simulink model "simulink_sketch"  (R2025b)
settings: Solver=VariableStepAuto  StartTime=0.0  StopTime=5  FixedStep=1e-6  MaxStep=1e-5  RelTol=1e-4
values from neighbouring files (symbols this model uses):
  bb_Cb = 1e-4    (= 0.0001)    [Akobel.m]
  bb_L2 = 1e-3    (= 0.001)    [Akobel.m]
  bb_R2 = 0.1    [Akobel.m]
  bb_series_R = 0.01    [Akobel.m]
  boost_Cdc = 2200e-6    (= 0.0022)    [Akobel.m]
  boost_Fsw = 10000    [Akobel.m]
  boost_L1 = 200e-6    (= 0.0002)    [Akobel.m]
  boost_R1 = 0.5    [Akobel.m]
  cc_Ib_trim_max = 0.5    [Akobel.m]
  cc_Iff_max = 1    [Akobel.m]
  cc_Ki = 0.02    [Akobel.m]
  cc_Kp = 0.002    [Akobel.m]
  cc_Ts = 1e-3    (= 0.001)    [Akobel.m]
  cc_Vdc_ref = 150    [Akobel.m]
  grid_freq = 60    [Akobel.m]
  grid_Ls1 = 0.05    [Akobel.m]
  grid_Rs1 = 5    [Akobel.m]
  grid_Vrms_test = 30.3    [Akobel.m]
  mppt_dD = 0.001    [Akobel.m]
  mppt_Dold_init = 0.75    [Akobel.m]
  mppt_filter_alpha = 0.1    [Akobel.m]
  mppt_max_duty_step = 0.02    [Akobel.m]
  mppt_Ts = 0.1    [Akobel.m]
  mppt_Vdc_hyst = 15    [Akobel.m]
  mppt_Vdc_start_clamp = 220    [Akobel.m]
  mppt_Vdc_trip = 280    [Akobel.m]
  pv_Cpv = 1000e-6    (= 0.001)    [Akobel.m]
  pv_irradiance = 1000    [Akobel.m]
  pv_temperature = 25    [Akobel.m]
  pwm_dt_deadtime_frac = 0.02    [Akobel.m]
  Ts = 1e-6    (= 1e-06)    [Akobel.m]
  xfmr_L_pu = 0.08    [Akobel.m]
  xfmr_R_pu = 0.002    [Akobel.m]
  xfmr_Sn_test = 5000    [Akobel.m]
  xfmr_V_test = grid_Vrms_test    (= 30.3)    [Akobel.m]
undefined symbols (not defined in the file or in its folder): Ion, Lithium
libraries: spsSeriesRLCBranchLib x11, spsIGBTLib x3, spsVoltageMeasurementLib x3, spsThreePhaseTransformerTwoWindingsLib x2, spsThreePhaseVIMeasurementLib x2, spsabctodq0Lib x2, spsPVArrayLib x1, spsDiodeLib x1, spsPWMGeneratorDCDCLib x1, spsBatteryLib x1, spsCurrentMeasurementLib x1, slpidlib x1
settings Model: Creator=inspiredkhalid  LastModifiedBy=inspiredkhalid

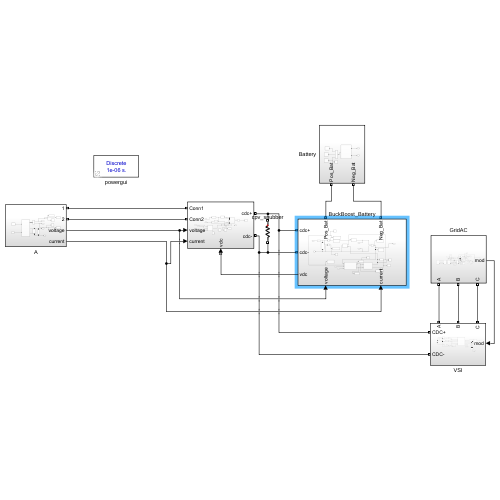
[thumbnail: Simulink's stored preview of the top-level diagram]
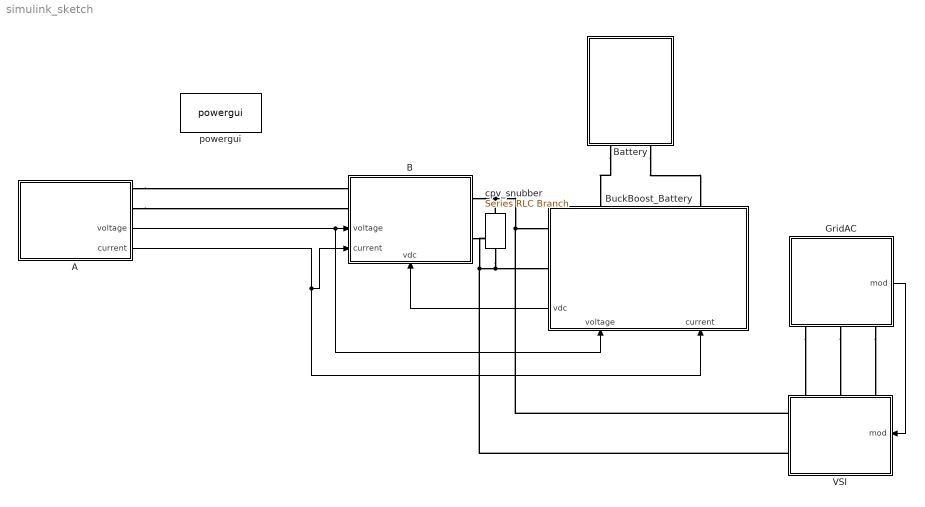
== system simulink_sketch ==
  A : Subsystem
      settings: PortSchema="{\"entries\":[{\"content\":{\"sides\":[{\"content\":{\"connectorIds\":[\"LConn1\",\"LConn2\",\"Out1\",\"Out2\"]},\"type\":\"ConnectorPlacement.EquallySpacedRectSide\",\"uuid\":\"f211f14f-7a8f-4763-b05c-a6f88137a125\"},{\"content\":{\"side\":\"RIGHT\"},\"type\":\"ConnectorPlacement.EquallySpacedRectSide\",\"uuid\":\"e9ab2bdb-56c2-498f-9900-91b8c83bb3bf\"},{\"content\":{\"side\":\"TOP\"},\"type\":\"ConnectorPlacement.EquallySpacedRectSide\",\"uuid\":\"9658df41-4415-4477-a305-d7a4a909d21d\"}]},\"type\":\"ConnectorPlacement.EquallySpacedConnector\",\"uuid\":\"93cd9b4f-abff-4e5b-becd-fd9ccd35f506\"}],\"packageUris\":[\"http://schema.mathworks.com/mf0/Connector/R2020b\"],\"version\":\"1.0\"}"
  B : Subsystem
      settings: PortSchema="{\"entries\":[{\"content\":{\"sides\":[{\"content\":{\"connectorIds\":[\"LConn1\",\"LConn2\",\"In1\",\"In2\"]},\"type\":\"ConnectorPlacement.EquallySpacedRectSide\",\"uuid\":\"2c74bd10-6af3-4400-a464-dc7b524de7bc\"},{\"content\":{\"connectorIds\":[\"RConn1\",\"RConn2\"],\"side\":\"RIGHT\"},\"type\":\"ConnectorPlacement.EquallySpacedRectSide\",\"uuid\":\"2332b9a4-ab65-4706-ac57-b493608de98d\"},{\"content\":{\"side\":\"TOP\"},\"type\":\"ConnectorPlacement.EquallySpacedRectSide\",\"uuid\":\"08936932-a96a-45d1-98bb-32320382a546\"},{\"content\":{\"connectorIds\":[\"In3\"],\"side\":\"BOTTOM\"},\"type\":\"ConnectorPlacement.EquallySpacedRectSide\",\"uuid\":\"91c62649-3be4-45ba-823f-24070183a03c\"}]},\"type\":\"ConnectorPlacement.EquallySpacedConnector\",\"uuid\":\"dd4d78f7-b16e-4c87-9b75-8b7f6c567d0f\"}],\"packageUris\":[\"http://schema.mathworks.com/mf0/Connector/R2020b\"],\"version\":\"1.0\"}"
  Battery : Subsystem
  BuckBoost_Battery : Subsystem
      settings: PortSchema="{\"entries\":[{\"content\":{\"sides\":[{\"content\":{\"connectorIds\":[\"LConn1\",\"LConn2\",\"Out1\"]},\"type\":\"ConnectorPlacement.EquallySpacedRectSide\",\"uuid\":\"f93f69dc-e0e8-4b3b-b6b4-88ae3b484cff\"},{\"content\":{\"side\":\"RIGHT\"},\"type\":\"ConnectorPlacement.EquallySpacedRectSide\",\"uuid\":\"d4d371e4-42d2-43a6-afc5-84f5672632c6\"},{\"content\":{\"connectorIds\":[\"LConn3\",\"LConn4\"],\"side\":\"TOP\"},\"type\":\"ConnectorPlacement.EquallySpacedRectSide\",\"uuid\":\"e974a5fd-4eac-4186-a4eb-b23fa22bd489\"},{\"content\":{\"connectorIds\":[\"In1\",\"In2\"],\"side\":\"BOTTOM\"},\"type\":\"ConnectorPlacement.EquallySpacedRectSide\",\"uuid\":\"43f62b17-f635-484f-a5a6-171bca4f90c5\"}]},\"type\":\"ConnectorPlacement.EquallySpacedConnector\",\"uuid\":\"5809b13c-41bb-4ec0-82ec-d14e3925591c\"}],\"packageUris\":[\"http://schema.mathworks.com/mf0/Connector/R2020b\"],\"version\":\"1.0\"}"
  GridAC : Subsystem
      settings: PortSchema="{\"entries\":[{\"content\":{\"sides\":[{\"content\":{\"connectorIds\":[\"LConn1\",\"LConn2\",\"LConn3\"]},\"type\":\"ConnectorPlacement.EquallySpacedRectSide\",\"uuid\":\"3c987b56-a6b3-414e-b913-46587328810b\"},{\"content\":{\"side\":\"RIGHT\"},\"type\":\"ConnectorPlacement.EquallySpacedRectSide\",\"uuid\":\"1ec4b9e6-98cb-4cc1-90b6-8ab385f8f2f7\"},{\"content\":{\"side\":\"TOP\"},\"type\":\"ConnectorPlacement.EquallySpacedRectSide\",\"uuid\":\"b7b4a685-ea9b-46c2-8886-60b08f7e650a\"},{\"content\":{\"connectorIds\":[\"Out1\"],\"side\":\"BOTTOM\"},\"type\":\"ConnectorPlacement.EquallySpacedRectSide\",\"uuid\":\"b927fc5e-4a89-4d3a-b035-fb59abf1a3eb\"}]},\"type\":\"ConnectorPlacement.EquallySpacedConnector\",\"uuid\":\"54d967a0-43e0-4c22-a5e9-acbfdfa3b599\"}],\"packageUris\":[\"http://schema.mathworks.com/mf0/Connector/R2020b\"],\"version\":\"1.0\"}"
  VSI : Subsystem
      settings: PortSchema="{\"entries\":[{\"content\":{\"sides\":[{\"content\":{\"connectorIds\":[\"LConn1\",\"LConn2\"]},\"type\":\"ConnectorPlacement.EquallySpacedRectSide\",\"uuid\":\"0ad929f8-4e0a-4843-968e-c440a9c9ffbc\"},{\"content\":{\"connectorIds\":[\"In1\"],\"side\":\"RIGHT\"},\"type\":\"ConnectorPlacement.EquallySpacedRectSide\",\"uuid\":\"290a1bb2-48c9-4171-842f-72ceda1cf966\"},{\"content\":{\"connectorIds\":[\"LConn3\",\"LConn4\",\"LConn5\"],\"side\":\"TOP\"},\"type\":\"ConnectorPlacement.EquallySpacedRectSide\",\"uuid\":\"ba767543-8593-4ea5-9207-7c4fa7bb7e96\"}]},\"type\":\"ConnectorPlacement.EquallySpacedConnector\",\"uuid\":\"5f02dbb0-dd03-4498-be26-732ab3bb6aa9\"}],\"packageUris\":[\"http://schema.mathworks.com/mf0/Connector/R2020b\"],\"version\":\"1.0\"}"
  cpv_snubber : spsSeriesRLCBranchLib/Series RLC Branch  LConnTagsString=__new0  RConnTagsString=__new0  BranchType=R  Resistance=1000  Inductance=boost_L1  SetiL0=off  InitialCurrent=0  Capacitance=1000e-6  Setx0=off  InitialVoltage=0  Measurements=None
  powergui : sps_lib/powergui  Priority=1  SimulationMode=Discrete  SampleTime=Ts  frequency=60  Iterations=50  frequencyindice=0  Pbase=100e6  ErrMax=1e-4  UnitsV=kV  UnitsW=MW  buscounter=0  FunctionMessages=off  echomessages=off  EnableUseOfTLC=off  CurrentSourceSwitches=off  DisableSnubberDevices=off  DisableRonSwitches=off  DisableVfSwitches=off  DisplayEquations=off  AutomaticDiscreteSolvers=off  SolverType=Backward Euler  Interpol=off  ExternalGateDelay=off  methode=off  Ts=Ts  x0status=blocks  SPID=on  SwTol=0  HookPort=off  NonlinearTolerance=1e-4  nMaxIteration=100  ContinueOnMaxIteration=off  RestoreLinks=warning  ResistiveCurrentMeasurement=off  Frange=[0:2:500]  Ylog=off  Xlog=on  ShowGrid=off  save=off  variable=ZData  structure=0  ZoomFFT=off  StartTime=0.0  cycles=1  DisplayStyle=1  fundamental=60  FreqAxis=off  MaxFrequency=1000  frequencyindicesteady=1  RmsSteady=1  display=off
  wires:
  A/1(voltage) -> BuckBoost_Battery/1(voltage), B/1(voltage)
  A/2(current) -> BuckBoost_Battery/2(current), B/2(current)
  GridAC/1(mod) -> VSI/1(mod)
  BuckBoost_Battery/1(vdc) -> B/3(vdc)
  connections:
  A/LConn1 -- B/LConn1
  A/LConn2 -- B/LConn2
  Battery/RConn1 -- BuckBoost_Battery/LConn3
  Battery/RConn2 -- BuckBoost_Battery/LConn4
  B/RConn1 -- VSI/LConn1 -- BuckBoost_Battery/LConn1 -- cpv_snubber/LConn1
  B/RConn2 -- VSI/LConn2 -- BuckBoost_Battery/LConn2 -- cpv_snubber/RConn1
  GridAC/LConn1 -- VSI/LConn3
  GridAC/LConn2 -- VSI/LConn4
  GridAC/LConn3 -- VSI/LConn5

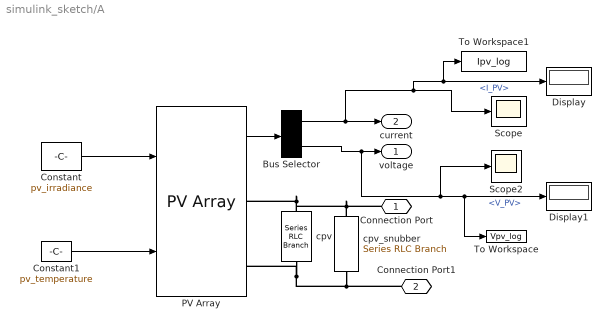
== system simulink_sketch/A ==
  Bus Selector : BusSelector  OutputSignals=I_PV,V_PV
  Constant : Constant  Value=pv_irradiance
  Constant1 : Constant  Value=pv_temperature
  Display : Display
  Display1 : Display
  PV Array : spsPVArrayLib/PV Array  Npar=pv_Npar  Nser=pv_Nser  PlotType=array @ 1000 W/m2 & specified temperatures  S_vec="[ 1000  500  100 ]"  Temp_C_vec="[ 45 25  ]"  ModuleName=User-defined  PlotWhenSelected=off  Pm=213.15  Ncell=60  Voc=36.3  Isc=7.84  Vm=29  Im=7.35  beta_Voc_pc=-0.36099  alpha_Isc_pc=0.102  beta_Voc=-0.13104  alpha_Isc=0.0079968  IL=7.8654  I0=2.9273e-10  nI=0.98119  Rsh=313.0553  Rs=0.39381  RobustModel=off  RobustCellTemperature=313.3991  BAL=on  Tc=1e-6  Tfilter=5e-5
  Scope : Scope
      settings: ActiveDisplayYMinimum=7.7837777500784995  ActiveDisplayYMaximum=7.87391809285628
  Scope2 : Scope
      settings: ActiveDisplayYMinimum=-2.4163883355478859  ActiveDisplayYMaximum=21.826134444811498  DataLoggingVariableName=ScopeData7
  To Workspace : ToWorkspace  VariableName=Vpv_log  SaveFormat=Timeseries  SampleTime=-1
  To Workspace1 : ToWorkspace  VariableName=Ipv_log  SaveFormat=Timeseries  SampleTime=-1
  cpv : spsSeriesRLCBranchLib/Series RLC Branch  LConnTagsString=__new0  RConnTagsString=__new0  BranchType=C  Resistance=1  Inductance=1e-3  SetiL0=off  InitialCurrent=0  Capacitance=pv_Cpv  Setx0=off  InitialVoltage=0  Measurements=None
  cpv_snubber : spsSeriesRLCBranchLib/Series RLC Branch  LConnTagsString=__new0  RConnTagsString=__new0  BranchType=RC  Resistance=8  Inductance=boost_L1  SetiL0=off  InitialCurrent=0  Capacitance=1000e-6  Setx0=off  InitialVoltage=0  Measurements=None
  Connection Port : PMIOPort  Side=Left
  Connection Port1 : PMIOPort  Port=2  Side=Left
  voltage : Outport
  current : Outport  Port=2
  wires:
  Constant/1 -> PV Array/1
  Constant1/1 -> PV Array/2
  PV Array/1 -> Bus Selector/1
  Bus Selector/2 -> To Workspace/1, Display1/1, Scope2/1, voltage/1  "<V_PV>"
  Bus Selector/1 -> To Workspace1/1, Display/1, Scope/1, current/1  "<I_PV>"
  connections:
  Connection Port/RConn1 -- cpv_snubber/LConn1 -- cpv/LConn1 -- PV Array/RConn1
  Connection Port1/RConn1 -- cpv_snubber/RConn1 -- cpv/RConn1 -- PV Array/RConn2

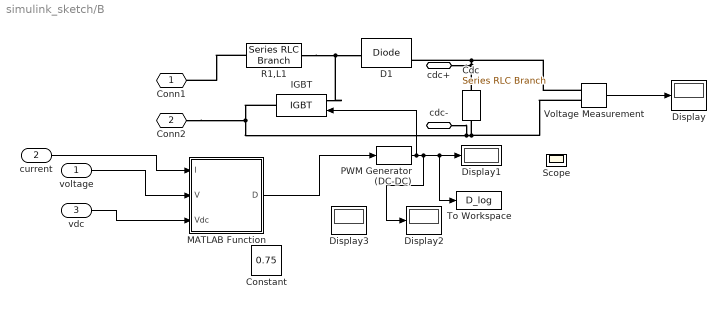
== system simulink_sketch/B ==
  voltage : Inport
  current : Inport  Port=2
  vdc : Inport  Port=3
  Cdc : spsSeriesRLCBranchLib/Series RLC Branch  LConnTagsString=__new0  RConnTagsString=__new0  BranchType=C  Resistance=1  Inductance=1e-3  SetiL0=off  InitialCurrent=0  Capacitance=boost_Cdc  Setx0=off  InitialVoltage=0  Measurements=None
  Constant : Constant  Value=0.75
  D1 : spsDiodeLib/Diode  Ron=0.001  Lon=0  Vf=0.8  IC=0  UseSnubber=1  Rs=500  Cs=250e-9  Measurements=on
  Display{,1..3} (4 alike) : Display
  "IGBT " : spsIGBTLib/IGBT  Ron=0.001  Lon=0  Vf=1  Tf=1e-6  Tt=2e-6  IC=0  Rs=1000  Cs=0.1e-6  Measurements=off
  MATLAB Function : MATLAB Function  TreatAsAtomicUnit=on  SystemSampleTime=mppt_Ts
  PWM Generator (DC-DC) : spsPWMGeneratorDCDCLib/PWM Generator (DC-DC)  Fsw=boost_Fsw  Ts=Ts
  R1,L1 : spsSeriesRLCBranchLib/Series RLC Branch  LConnTagsString=__new0  RConnTagsString=__new0  BranchType=RL  Resistance=boost_R1  Inductance=boost_L1  SetiL0=off  InitialCurrent=0  Capacitance=1e-6  Setx0=off  InitialVoltage=0  Measurements=None
  Scope : Scope
      settings: ActiveDisplayYMinimum=-1  ActiveDisplayYMaximum=1
  To Workspace : ToWorkspace  VariableName=D_log  SaveFormat=Timeseries  SampleTime=-1
  Voltage Measurement : spsVoltageMeasurementLib/Voltage Measurement  PhasorSimulation=off  OutputType=Complex  PSBequivalent=0
  Conn1 : PMIOPort  Side=Left
  Conn2 : PMIOPort  Port=2  Side=Left
  cdc+ : PMIOPort  Port=3  Side=Right
  cdc- : PMIOPort  Port=4  Side=Right
  wires:
  Voltage Measurement/1 -> Display/1
  PWM Generator (DC-DC)/1 -> Display2/1, To Workspace/1, Display1/1, "IGBT "/1
  voltage/1 -> MATLAB Function/2(V)
  current/1 -> MATLAB Function/1(I)
  vdc/1 -> MATLAB Function/3(Vdc)
  MATLAB Function/1(D) -> PWM Generator (DC-DC)/1
  connections:
  R1,L1/LConn1 -- Conn1/RConn1
  Conn2/RConn1 -- cdc-/RConn1 -- Voltage Measurement/LConn2 -- Cdc/RConn1 -- "IGBT "/RConn1
  Cdc/LConn1 -- cdc+/RConn1 -- Voltage Measurement/LConn1 -- D1/RConn1
  R1,L1/RConn1 -- "IGBT "/LConn1 -- D1/LConn1

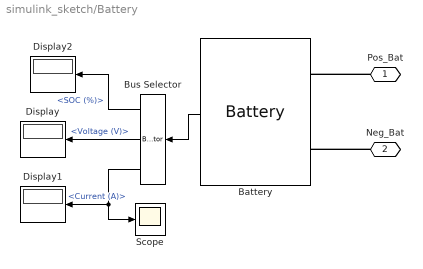
== system simulink_sketch/Battery ==
  Battery : spsBatteryLib/Battery  BatType=Lithium-Ion  NomV=batt_nominal_voltage  NomQ=batt_rated_capacity  SOC=100  Batt_Tr=30  PresetModel=on  MaxQ=100  MinV=36  FullV=55.8714  Dis_rate=43.4783  R=0.0048  Normal_OP=90.4348  expZone="[51.8585      4.91304]"
  Bus Selector : BusSelector  OutputSignals=SOC (%),Voltage (V),Current (A)
  Display : Display
  Display1 : Display
  Display2 : Display
  Scope : Scope
      settings: DataLoggingVariableName=ScopeData13
  Pos_Bat : PMIOPort  Side=Right
  Neg_Bat : PMIOPort  Port=2  Side=Right
  wires:
  Battery/1 -> Bus Selector/1
  Bus Selector/2 -> Display/1  "<Voltage (V)>"
  Bus Selector/1 -> Display2/1  "<SOC (%)>"
  Bus Selector/3 -> Scope/1, Display1/1  "<Current (A)>"
  connections:
  Pos_Bat/RConn1 -- Battery/LConn1
  Neg_Bat/RConn1 -- Battery/LConn2

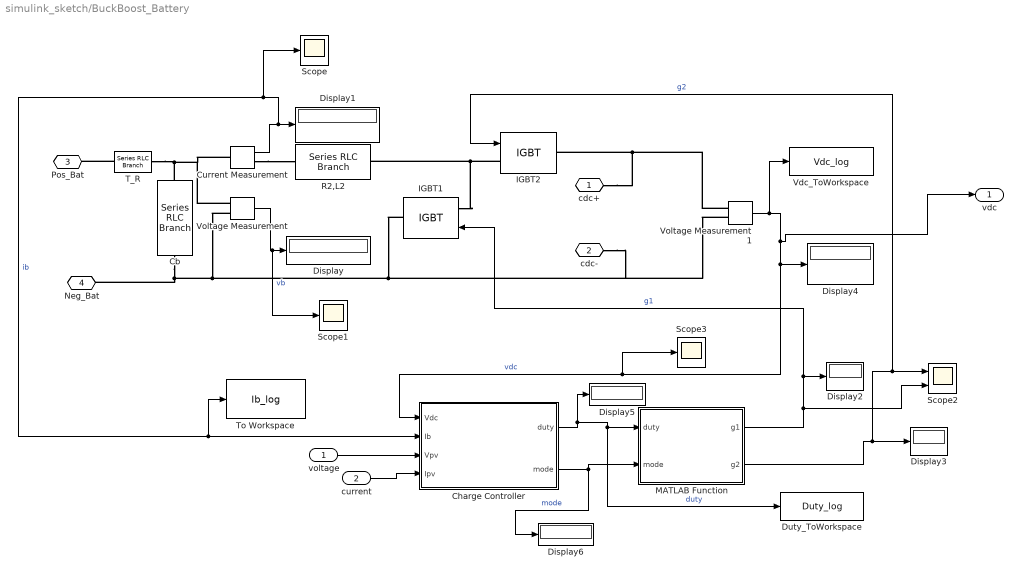
== system simulink_sketch/BuckBoost_Battery ==
  voltage : Inport
  current : Inport  Port=2
  Cb : spsSeriesRLCBranchLib/Series RLC Branch  LConnTagsString=__new0  RConnTagsString=__new0  BranchType=C  Resistance=1  Inductance=1e-3  SetiL0=off  InitialCurrent=0  Capacitance=bb_Cb  Setx0=off  InitialVoltage=0  Measurements=None
  "Charge Controller " : MATLAB Function  TreatAsAtomicUnit=on  SystemSampleTime=cc_Ts
  Current Measurement : spsCurrentMeasurementLib/Current Measurement  PhasorSimulation=off  OutputType=Complex  PSBequivalent=0
  Display{,1..6} (7 alike) : Display
  Duty_ToWorkspace : ToWorkspace  VariableName=Duty_log  SaveFormat=Timeseries  SampleTime=-1
  "IGBT1  " : spsIGBTLib/IGBT  Ron=0.001  Lon=0  Vf=1  Tf=1e-6  Tt=2e-6  IC=0  Rs=500  Cs=250e-9  Measurements=off
  "IGBT2 " : spsIGBTLib/IGBT  Ron=0.001  Lon=0  Vf=1  Tf=1e-6  Tt=2e-6  IC=0  Rs=500  Cs=250e-9  Measurements=off
  MATLAB Function : MATLAB Function  TreatAsAtomicUnit=on  SystemSampleTime=Ts
  R2,L2 : spsSeriesRLCBranchLib/Series RLC Branch  LConnTagsString=__new0  RConnTagsString=__new0  BranchType=RL  Resistance=bb_R2  Inductance=bb_L2  SetiL0=off  InitialCurrent=0  Capacitance=1e-6  Setx0=off  InitialVoltage=0  Measurements=None
  Scope : Scope
      settings: ActiveDisplayYMinimum=-1.6642908059310153  ActiveDisplayYMaximum=14.289691482318968  DataLoggingVariableName=ScopeData2
  Scope1 : Scope
      settings: DataLoggingVariableName=ScopeData3
  Scope2 : Scope  NumInputPorts=2
      settings: DataLoggingVariableName=ScopeData4
  Scope3 : Scope
      settings: ActiveDisplayYMinimum=-7.5370517682941776  ActiveDisplayYMaximum=68.122712038628222  DataLoggingVariableName=ScopeData5
  T_R : spsSeriesRLCBranchLib/Series RLC Branch  LConnTagsString=__new0  RConnTagsString=__new0  BranchType=R  Resistance=bb_series_R  Inductance=1e-3  SetiL0=off  InitialCurrent=0  Capacitance=1e-6  Setx0=off  InitialVoltage=0  Measurements=None
  To Workspace : ToWorkspace  VariableName=Ib_log  SaveFormat=Timeseries  SampleTime=-1
  Vdc_ToWorkspace : ToWorkspace  VariableName=Vdc_log  SaveFormat=Timeseries  SampleTime=-1
  Voltage Measurement : spsVoltageMeasurementLib/Voltage Measurement  PhasorSimulation=off  OutputType=Complex  PSBequivalent=0
  Voltage Measurement1 : spsVoltageMeasurementLib/Voltage Measurement  PhasorSimulation=off  OutputType=Complex  PSBequivalent=0
  cdc+ : PMIOPort  Side=Left
  cdc- : PMIOPort  Port=2  Side=Left
  Pos_Bat : PMIOPort  Port=3  Side=Left
  Neg_Bat : PMIOPort  Port=4  Side=Left
  vdc : Outport
  wires:
  Voltage Measurement/1 -> Scope1/1, Display/1  "vb"
  Current Measurement/1 -> To Workspace/1, "Charge Controller "/2(Ib), Scope/1, Display1/1  "ib"
  Voltage Measurement1/1 -> Vdc_ToWorkspace/1, vdc/1, Display4/1, Scope3/1, "Charge Controller "/1(Vdc)  "vdc"
  "Charge Controller "/1(duty) -> Duty_ToWorkspace/1, MATLAB Function/1(duty), Display5/1  "duty"
  "Charge Controller "/2(mode) -> MATLAB Function/2(mode), Display6/1  "mode"
  MATLAB Function/1(g1) -> Display2/1, "IGBT1  "/1, Scope2/2  "g1"
  MATLAB Function/2(g2) -> Display3/1, "IGBT2 "/1, Scope2/1  "g2"
  current/1 -> "Charge Controller "/4(Ipv)
  voltage/1 -> "Charge Controller "/3(Vpv)
  connections:
  "IGBT2 "/LConn1 -- R2,L2/RConn1 -- "IGBT1  "/LConn1
  T_R/RConn1 -- Voltage Measurement/LConn1 -- Current Measurement/LConn1 -- Cb/LConn1
  T_R/LConn1 -- Pos_Bat/RConn1
  Current Measurement/RConn1 -- R2,L2/LConn1
  Voltage Measurement1/LConn1 -- cdc+/RConn1 -- "IGBT2 "/RConn1
  "IGBT1  "/RConn1 -- cdc-/RConn1 -- Voltage Measurement1/LConn2 -- Voltage Measurement/LConn2 -- Cb/RConn1 -- Neg_Bat/RConn1

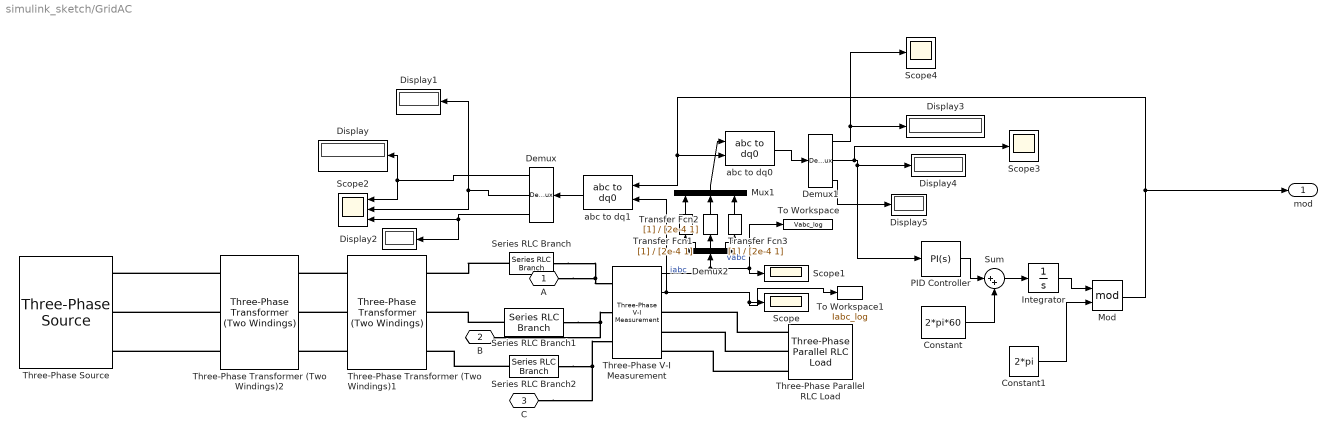
== system simulink_sketch/GridAC ==
  Constant : Constant  Value=2*pi*60
  Constant1 : Constant  Value=2*pi
  Demux : Demux  Outputs=3
  Demux1 : Demux  Outputs=3
  Demux2 : Demux  Outputs=3
  Display{,1..5} (6 alike) : Display
  Integrator : Integrator
  Mod : Math  Operator=mod
  Mux1 : Mux  Inputs=3
  PID Controller : slpidlib/PID Controller  Controller=PI  Form=Parallel  TimeDomain=Continuous-time  UseExternalTs=off  SampleTime=-1  IntegratorMethod=Forward Euler  FilterMethod=Forward Euler  ControllerParametersSource=internal  P=-0.05  I=-0.1  UseKiTs=off  D=0  UseExternalDerivativeSource=off  N=100  UseFilter=on  TunerSelectOption=Transfer Function Based (PID Tuner App)  InitialConditionSource=internal  InitialConditionForIntegrator=0  InitialConditionForFilter=0  DifferentiatorICPrevScaledInput=0  ExternalReset=none  TrackingMode=off  Kt=1  LimitOutput=on  SatLimitsSource=internal  UpperSaturationLimit=20  LowerSaturationLimit=-20  LinearizeAsGain=on  AntiWindupMode=clamping  Kb=1  LimitIntegrator=off  UpperIntegratorSaturationLimit=inf  LowerIntegratorSaturationLimit=-inf  POutMin=[]  POutMax=[]  IOutMin=[]  IOutMax=[]  DOutMin=[]  DOutMax=[]  NOutMin=[]  NOutMax=[]  SumOutMin=[]  SumOutMax=[]  SaturationOutMin=[]  SaturationOutMax=[]  PParamMin=[]  PParamMax=[]  IParamMin=[]  IParamMax=[]  DParamMin=[]  DParamMax=[]  NParamMin=[]  NParamMax=[]  KbParamMin=[]  KbParamMax=[]  KtParamMin=[]  KtParamMax=[]  KbOutMin=[]  KbOutMax=[]  KtOutMin=[]  KtOutMax=[]  IntegratorOutMin=[]  IntegratorOutMax=[]  FilterOutMin=[]  FilterOutMax=[]  SumI1OutMin=[]  SumI1OutMax=[]  SumI2OutMin=[]  SumI2OutMax=[]  SumI3OutMin=[]  SumI3OutMax=[]  SumI4OutMin=[]  SumI4OutMax=[]  SumDOutMin=[]  SumDOutMax=[]  DifferentiatorOutMin=[]  DifferentiatorOutMax=[]  FilterDiffOutCoefMin=[]  FilterDiffOutCoefMax=[]  ReciprocalOutMin=[]  ReciprocalOutMax=[]  SumDenOutMin=[]  SumDenOutMax=[]  SumNumOutMin=[]  SumNumOutMax=[]  DivideOutMin=[]  DivideOutMax=[]  UdiffTsProdOutMin=[]  UdiffTsProdOutMax=[]  NTsProdOutMin=[]  NTsProdOutMax=[]  UintegralTsProdOutMin=[]  UintegralTsProdOutMax=[]  UngainTsProdOutMin=[]  UngainTsProdOutMax=[]  ClampingZeroOutDataTypeStr=Inherit: Inherit via back propagation  ClampingZeroOutMin=[]  ClampingZeroOutMax=[]  FilterDenConstantOutDataTypeStr=Inherit: Inherit via back propagation  FilterDenConstantOutMin=[]  FilterDenConstantOutMax=[]  PCopyOutDataTypeStr=Inherit: Inherit via back propagation  PCopyOutMin=[]  PCopyOutMax=[]  NCopyOutDataTypeStr=Inherit: Inherit via back propagation  NCopyOutMin=[]  NCopyOutMax=[]  IntegratorContinuousStateAttributes=''  IntegratorStateMustResolveToSignalObject=off  IntegratorRTWStateStorageClass=Auto  FilterContinuousStateAttributes=''  FilterStateMustResolveToSignalObject=off  FilterRTWStateStorageClass=Auto  ParallelPVariant=InternalParameters  IdealPVariant=Disabled  IVariant=InternalParameters  DVariant=InternalParameters  IntegratorVariant=Continuous  SatVariant=Disabled  AWVariant=Passthrough  PCopyVariant=Disabled  TRVariant=Disabled  FdbkBlocksVariant=Forward  IdealPFdbkVariant=Disabled  SatFdbkVariant=Disabled  DerivativeFilterVariant=ContFilter  NVariant=InternalParameters  NCopyVariant=Disabled  FilterICVariant=InternalICsFilter  IntegratorICVariant=InternalICs  ExternalResetVariant=Disabled  TRSumVariant=Passthrough  SumFdbkVariant=Disabled  SumVariant=Sum_PID  TsampFilterVariant=InternalTs  TsampNgainVariant=Passthrough  TsampIntegralVariant=Passthrough  ExternalSaturationOutDataTypeStr=Inherit: Same as second input  DerivativeSourceVariant=ErrorSignal  PreIntVariant=InternalPreInt
  Scope{,1,3..4} (4 alike) : Scope
      Scope settings: ActiveDisplayYMinimum=-1.7996046557008947  ActiveDisplayYMaximum=2.5741007420430475  DataLoggingVariableName=ScopeData6
      Scope1 settings: ActiveDisplayYMinimum=-407.48253485429876  ActiveDisplayYMaximum=407.48253511631697  DataLoggingVariableName=ScopeData8
      Scope3 settings: ActiveDisplayYMinimum=-1  ActiveDisplayYMaximum=1  DataLoggingVariableName=ScopeData11
      Scope4 settings: ActiveDisplayYMinimum=-1563.9504384708348  ActiveDisplayYMaximum=1752.8134943632215  DataLoggingVariableName=ScopeData12
  Scope2 : Scope  NumInputPorts=3
      settings: ActiveDisplayYMinimum=-469.29997145914172  ActiveDisplayYMaximum=482.438808919499  DataLoggingVariableName=ScopeData10
  Series RLC Branch : spsSeriesRLCBranchLib/Series RLC Branch  LConnTagsString=__new0  RConnTagsString=__new0  BranchType=RL  Resistance=grid_Rs1  Inductance=grid_Ls1  SetiL0=off  InitialCurrent=0  Capacitance=1e-6  Setx0=off  InitialVoltage=0  Measurements=None
  Series RLC Branch1 : spsSeriesRLCBranchLib/Series RLC Branch  LConnTagsString=__new0  RConnTagsString=__new0  BranchType=RL  Resistance=grid_Rs1  Inductance=grid_Ls1  SetiL0=off  InitialCurrent=0  Capacitance=1e-6  Setx0=off  InitialVoltage=0  Measurements=None
  Series RLC Branch2 : spsSeriesRLCBranchLib/Series RLC Branch  LConnTagsString=__new0  RConnTagsString=__new0  BranchType=RL  Resistance=grid_Rs1  Inductance=grid_Ls1  SetiL0=off  InitialCurrent=0  Capacitance=1e-6  Setx0=off  InitialVoltage=0  Measurements=None
  Sum : Sum  Inputs=|++
  Three-Phase Parallel RLC Load : spsThreePhaseParallelRLCLoadLib/Three-Phase Parallel RLC Load  LConnTagsString=A|B|C  Configuration=Y (grounded)  NominalVoltage=300  Vabc=[1e3 1e3 1e3]  Vabcp=[1e3 1e3 1e3]  NominalFrequency=60  UnbalancedPower=off  ActivePower=100  InductivePower=100  CapacitivePower=100  Pabc=[10e3 9e3 11e3]  QLabc=[100 90 110]  QCabc=[100 90 110]  Pabcp=[10e3 9e3 11e3]  QLabcp=[100 90 110]  QCabcp=[100 90 110]  Measurements=None  LoadType=constant Z
  Three-Phase Transformer (Two Windings)1 : spsThreePhaseTransformerTwoWindingsLib/Three-Phase Transformer (Two Windings)  Winding1Connection=Yg  Winding2Connection=Yg  CoreType=Three single-phase transformers  SetSaturation=off  Hysteresis=off  DataFile='hysteresis'  SetInitialFlux=off  Measurements=None  UNITS=pu  NominalPower=[ xfmr_Sn_test grid_freq]  Winding1=[ xfmr_V_test , xfmr_R_pu , xfmr_L_pu ]  Winding2=[ xfmr_V_test , xfmr_R_pu , xfmr_L_pu ]  Rm=500  Lm=500  L0=0.5  Saturation=[ 0,0 ; 0.0024,1.2 ; 1.0,1.52 ]  InitialFluxes=[ 0.8 , -0.8 , 0.7 ]  BreakLoop=off  DiscreteSolver=Trapezoidal iterative  DataType=off  TransfoNumber=1
  Three-Phase Transformer (Two Windings)2 : spsThreePhaseTransformerTwoWindingsLib/Three-Phase Transformer (Two Windings)  Winding1Connection=Yg  Winding2Connection=Yg  CoreType=Three single-phase transformers  SetSaturation=off  Hysteresis=off  DataFile='hysteresis'  SetInitialFlux=off  Measurements=None  UNITS=pu  NominalPower=[ xfmr_Sn_test grid_freq]  Winding1=[ xfmr_V_test , xfmr_R_pu , xfmr_L_pu ]  Winding2=[ xfmr_V_test , xfmr_R_pu , xfmr_L_pu ]  Rm=500  Lm=500  L0=0.5  Saturation=[ 0,0 ; 0.0024,1.2 ; 1.0,1.52 ]  InitialFluxes=[ 0.8 , -0.8 , 0.7 ]  BreakLoop=off  DiscreteSolver=Trapezoidal iterative  DataType=off  TransfoNumber=1
  Three-Phase V-I Measurement : spsThreePhaseVIMeasurementLib/Three-Phase V-I Measurement  VoltageMeasurement=phase-to-ground  SetLabelV=off  LabelV=Vabc  Vpu=off  VpuLL=off  CurrentMeasurement=yes  SetLabelI=off  LabelI=Iabc  Ipu=off  Pbase=100e6  Vbase=500e3  OutputType=Complex  PhasorSimulation=off  PSBequivalent=0
  Three-Phase Source : spsThreePhaseSourceLib/Three-Phase Source  InternalConnection=Yg  VoltagePhases=on  Voltage=400  PhaseAngle=0  Voltage_phases=[grid_Vrms_test grid_Vrms_test grid_Vrms_test]/sqrt(3)  PhaseAngles_phases=[0 -120 +120]  Frequency=60  NonIdealSource=on  SpecifyImpedance=off  Resistance=0.000229  Inductance=4.25e-6  ShortCircuitLevel=100e6  BaseVoltage=400  XRratio=7  BusType=swing  Pref=10e3  Qref=0  Prefabc=[10e3, 10e3, 10e3]  Qrefabc=[0, 0, 0]  Qmin=-inf  Qmax=inf
  To Workspace : ToWorkspace  VariableName=Vabc_log  SaveFormat=Timeseries  SampleTime=-1
  To Workspace1 : ToWorkspace  VariableName=Iabc_log  SaveFormat=Timeseries  SampleTime=-1
  Transfer Fcn1 : TransferFcn  Denominator=[2e-4 1]
  Transfer Fcn2 : TransferFcn  Denominator=[2e-4 1]
  Transfer Fcn3 : TransferFcn  Denominator=[2e-4 1]
  abc to dq0 : spsabctodq0Lib/abc to dq0  Alignment=90 degrees behind phase A axis
  abc to dq1 : spsabctodq0Lib/abc to dq0  Alignment=90 degrees behind phase A axis
  A : PMIOPort  Side=Left
  B : PMIOPort  Port=2  Side=Left
  C : PMIOPort  Port=3  Side=Left
  mod : Outport
  wires:
  Three-Phase V-I Measurement/1 -> Scope1/1, To Workspace/1, Demux2/1  "vabc"
  Three-Phase V-I Measurement/2 -> abc to dq1/1, To Workspace1/1, Scope/1  "iabc"
  abc to dq1/1 -> Demux/1
  abc to dq0/1 -> Demux1/1
  Demux/2 -> Display1/1, Scope2/2
  Demux/3 -> Display2/1, Scope2/3
  Demux/1 -> Display/1, Scope2/1
  Demux1/1 -> Scope4/1, Display3/1
  Demux1/2 -> Scope3/1, PID Controller/1, Display4/1
  Demux1/3 -> Display5/1
  PID Controller/1 -> Sum/1
  Constant/1 -> Sum/2
  Sum/1 -> Integrator/1
  Integrator/1 -> Mod/1
  Constant1/1 -> Mod/2
  Demux2/1 -> Transfer Fcn1/1
  Demux2/2 -> Transfer Fcn2/1
  Demux2/3 -> Transfer Fcn3/1
  Transfer Fcn1/1 -> Mux1/1
  Transfer Fcn2/1 -> Mux1/2
  Transfer Fcn3/1 -> Mux1/3
  Mux1/1 -> abc to dq0/1
  Mod/1 -> abc to dq1/2, abc to dq0/2, mod/1
  connections:
  Three-Phase Transformer (Two Windings)2/LConn1 -- Three-Phase Source/RConn1
  Three-Phase Transformer (Two Windings)1/LConn1 -- Three-Phase Transformer (Two Windings)2/RConn1
  Series RLC Branch/LConn1 -- Three-Phase Transformer (Two Windings)1/RConn1
  Series RLC Branch/RConn1 -- A/RConn1 -- Three-Phase V-I Measurement/LConn1
  Series RLC Branch1/LConn1 -- Three-Phase Transformer (Two Windings)1/RConn2
  Series RLC Branch2/LConn1 -- Three-Phase Transformer (Two Windings)1/RConn3
  Three-Phase Transformer (Two Windings)1/LConn3 -- Three-Phase Transformer (Two Windings)2/RConn3
  Three-Phase Transformer (Two Windings)1/LConn2 -- Three-Phase Transformer (Two Windings)2/RConn2
  Three-Phase Transformer (Two Windings)2/LConn2 -- Three-Phase Source/RConn2
  Three-Phase Transformer (Two Windings)2/LConn3 -- Three-Phase Source/RConn3
  Series RLC Branch1/RConn1 -- Three-Phase V-I Measurement/LConn2 -- B/RConn1
  Series RLC Branch2/RConn1 -- C/RConn1 -- Three-Phase V-I Measurement/LConn3
  Three-Phase Parallel RLC Load/LConn2 -- Three-Phase V-I Measurement/RConn2
  Three-Phase Parallel RLC Load/LConn1 -- Three-Phase V-I Measurement/RConn1
  Three-Phase Parallel RLC Load/LConn3 -- Three-Phase V-I Measurement/RConn3

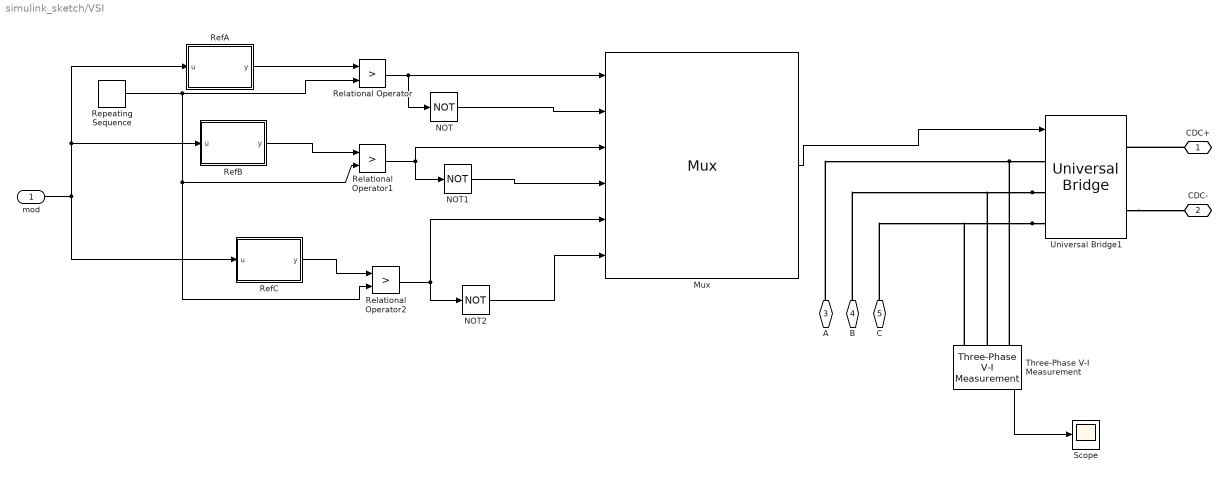
== system simulink_sketch/VSI ==
  mod : Inport
  Mux : Mux  Inputs=6
  NOT : Logic  Operator=NOT  IconShape=distinctive  AllPortsSameDT=off  OutDataTypeStr=boolean
  NOT1 : Logic  Operator=NOT  IconShape=distinctive  AllPortsSameDT=off  OutDataTypeStr=boolean
  NOT2 : Logic  Operator=NOT  IconShape=distinctive  AllPortsSameDT=off  OutDataTypeStr=boolean
  RefA : MATLAB Function  TreatAsAtomicUnit=on
  RefB : MATLAB Function  TreatAsAtomicUnit=on
  RefC : MATLAB Function  TreatAsAtomicUnit=on
  Relational Operator : RelationalOperator  Operator=>  OutDataTypeStr=boolean  RndMeth=Simplest  InputSameDT=off
  Relational Operator1 : RelationalOperator  Operator=>  OutDataTypeStr=boolean  RndMeth=Simplest  InputSameDT=off
  Relational Operator2 : RelationalOperator  Operator=>  OutDataTypeStr=boolean  RndMeth=Simplest  InputSameDT=off
  Repeating Sequence : simulink/Sources/Repeating Sequence  rep_seq_t=[0 0.00005 0.0001]  rep_seq_y=[-1 1 -1]
  Scope : Scope
      settings: ActiveDisplayYMinimum=-20.097502542386408  ActiveDisplayYMaximum=20.966890255539155  DataLoggingVariableName=ScopeData9
  Three-Phase V-I Measurement : spsThreePhaseVIMeasurementLib/Three-Phase V-I Measurement  VoltageMeasurement=phase-to-ground  SetLabelV=off  LabelV=Vabc  Vpu=off  VpuLL=off  CurrentMeasurement=yes  SetLabelI=off  LabelI=Iabc  Ipu=off  Pbase=100e6  Vbase=500e3  OutputType=Complex  PhasorSimulation=off  PSBequivalent=0
  Universal Bridge1 : spsUniversalBridgeLib/Universal Bridge  Arms=3  SnubberResistance=500  SnubberCapacitance=250e-9  Device=IGBT / Diodes  Ron=1e-3  Lon=0  ForwardVoltages="[  0  0  ]"  ForwardVoltage=0  GTOparameters=[ 10e-6 , 20e-6 ]  IGBTparameters=[ 1e-6 , 2e-6 ]  Measurements=None  Measurements_2=None  converterType=Rectifier
  CDC+ : PMIOPort  Side=Left
  CDC- : PMIOPort  Port=2  Side=Left
  A : PMIOPort  Port=3  Side=Left
  B : PMIOPort  Port=4  Side=Left
  C : PMIOPort  Port=5  Side=Left
  wires:
  RefA/1(y) -> Relational Operator/1
  RefB/1(y) -> Relational Operator1/1
  RefC/1(y) -> Relational Operator2/1
  Repeating Sequence/1 -> Relational Operator/2, Relational Operator1/2, Relational Operator2/2
  Relational Operator/1 -> Mux/1, NOT/1
  Relational Operator1/1 -> Mux/3, NOT1/1
  NOT/1 -> Mux/2
  NOT1/1 -> Mux/4
  Relational Operator2/1 -> NOT2/1, Mux/5
  NOT2/1 -> Mux/6
  Mux/1 -> Universal Bridge1/1
  Three-Phase V-I Measurement/1 -> Scope/1
  mod/1 -> RefC/1(u), RefB/1(u), RefA/1(u)
  connections:
  Three-Phase V-I Measurement/LConn1 -- A/RConn1 -- Universal Bridge1/LConn1
  Universal Bridge1/LConn2 -- B/RConn1 -- Three-Phase V-I Measurement/LConn2
  Universal Bridge1/LConn3 -- C/RConn1 -- Three-Phase V-I Measurement/LConn3
  CDC+/RConn1 -- Universal Bridge1/RConn1
  Universal Bridge1/RConn2 -- CDC-/RConn1

== matlab function simulink_sketch/BuckBoost_Battery/Charge Controller  ==
  data: Vdc input; duty output; Ib input; mode output; Vpv input; Ipv input; cc_Vdc_ref parameter; cc_Kp parameter; cc_Ki parameter; cc_Ib_trim_max parameter; cc_Iff_max parameter; cc_Ts parameter
function [duty, mode] = fcn(Vdc, Ib, Vpv, Ipv, cc_Vdc_ref, cc_Kp, cc_Ki, cc_Ib_trim_max, cc_Iff_max, cc_Ts)
persistent integ_v integ_i
if isempty(integ_v)
    integ_v = 0;
    integ_i = 0;
end

Ts_local = cc_Ts;

% Feed-forward
Ppv = Vpv * Ipv;
Iff = Ppv / cc_Vdc_ref;
Iff = min(max(Iff, -cc_Iff_max), cc_Iff_max);

% Outer loop: Vdc regulation
err_v = Vdc - cc_Vdc_ref;
integ_v = integ_v + err_v*Ts_local;
integ_v = min(max(integ_v, -2), 2);
Ib_trim = cc_Kp*err_v + cc_Ki*integ_v;
Ib_trim = min(max(Ib_trim, -cc_Ib_trim_max), cc_Ib_trim_max);

Ib_ref = Iff + Ib_trim;

% Inner loop: fast current tracking (not yet parameterized)
Kp_i = 0.05;
Ki_i = 0.5;
err_i = Ib_ref - Ib;
integ_i = integ_i + err_i*Ts_local;
integ_i = min(max(integ_i, -1), 1);
ctrl = Kp_i*err_i + Ki_i*integ_i;
ctrl = min(max(ctrl, -0.9), 0.9);

if ctrl > 0
    duty = max(ctrl, 0.1);
    mode = 1;
else
    duty = max(-ctrl, 0.1);
    mode = 0;
end

== matlab function simulink_sketch/B/MATLAB Function ==
  data: I input; V input; D output; Vdc input; mppt_dD parameter; mppt_filter_alpha parameter; mppt_Dold_init parameter; mppt_Vdc_start_clamp parameter; mppt_Vdc_trip parameter; mppt_Vdc_hyst parameter; mppt_max_duty_step parameter
function D = fcn(I, V, Vdc, mppt_dD, mppt_filter_alpha, mppt_Dold_init, mppt_Vdc_start_clamp, mppt_Vdc_trip, mppt_Vdc_hyst, mppt_max_duty_step)
    % Declare persistent variables (Added: clampActive and D_prev)
    persistent Pold Dold direction Vfilt Ifilt initialized clampActive D_prev
    
    % Initialization block
    if isempty(initialized)
        Pold = 0;
        Dold = mppt_Dold_init;
        direction = 1;
        Vfilt = V;
        Ifilt = I;
        clampActive = false;      % Initialize hysteresis flag to false
        D_prev = mppt_Dold_init;  % Initialize rate limiter history
        initialized = true;
    end
    
    % --- UPGRADE 1: HYSTERESIS ON THE CLAMP ---
    if Vdc > mppt_Vdc_start_clamp
        clampActive = true;
    elseif Vdc < (mppt_Vdc_start_clamp - mppt_Vdc_hyst)
        clampActive = false;
    end
    
    % Compute D_max based on the persistent clamp status
    if clampActive
        D_max = 0.9 - 0.8 * (Vdc - mppt_Vdc_start_clamp) / (mppt_Vdc_trip - mppt_Vdc_start_clamp);
        D_max = max(D_max, 0.1);
    else
        D_max = 0.9;
    end
    
    % Low-pass filtering of inputs
    Vfilt = mppt_filter_alpha * V + (1 - mppt_filter_alpha) * Vfilt;
    Ifilt = mppt_filter_alpha * I + (1 - mppt_filter_alpha) * Ifilt;
    
    % Perturb and Observe (P&O) Core Logic
    P = Vfilt * Ifilt;
    if P > Pold
        Dold = Dold + direction * mppt_dD;
    else
        direction = -direction;
        Dold = Dold + direction * mppt_dD;
    end
    
    % Keep the search state itself sane (internal memory)
    Dold = min(max(Dold, 0.1), 0.9); 
    Pold = P;
    
    % Target calculation (safety-clamped output before rate limiting)
    D_target = min(max(Dold, 0.1), D_max);
    
    % --- UPGRADE 2: RATE LIMITER ---
    % Cap the maximum step size to prevent hard slamming
    D = D_prev + max(min(D_target - D_prev, mppt_max_duty_step), -mppt_max_duty_step);
    
    % Save current duty cycle for the next time step
    D_prev = D;
end

== matlab function simulink_sketch/BuckBoost_Battery/MATLAB Function ==
  data: duty input; g1 output; mode input; g2 output; boost_Fsw parameter; Ts parameter; pwm_dt_deadtime_frac parameter
function [g1, g2] = fcn(duty, mode, boost_Fsw, Ts, pwm_dt_deadtime_frac)

persistent counter
if isempty(counter)
    counter = 0;
end

counter = counter + Ts*boost_Fsw;
if counter >= 1
    counter = counter - 1;
end

if mode >= 0.5
    if counter < duty - pwm_dt_deadtime_frac/2
        g2 = 1; g1 = 0;
    elseif counter > duty + pwm_dt_deadtime_frac/2
        g2 = 0; g1 = 1;
    else
        g2 = 0; g1 = 0;
    end
else
    if counter < duty - pwm_dt_deadtime_frac/2
        g1 = 1; g2 = 0;
    elseif counter > duty + pwm_dt_deadtime_frac/2
        g1 = 0; g2 = 1;
    else
        g1 = 0; g2 = 0;
    end
end

== matlab function simulink_sketch/VSI/RefA ==
  data: u input; y output
function y = fcn(u)

y = sin(u);

== matlab function simulink_sketch/VSI/RefB ==
  data: u input; y output
function y = fcn(u)

y = sin(u - 2*pi/3);

== matlab function simulink_sketch/VSI/RefC ==
  data: u input; y output
function y = fcn(u)

y = sin(u + 2*pi/3);
